simulink model "Control_PID_Senoidal_orientacion"  (R2024b)
settings: Solver=FixedStepAuto  StartTime=0.0  StopTime=30.0  FixedStep=1e-3  RelTol=1e-3
settings Model: Creator=Raul Robles  LastModifiedBy=Raul Robles

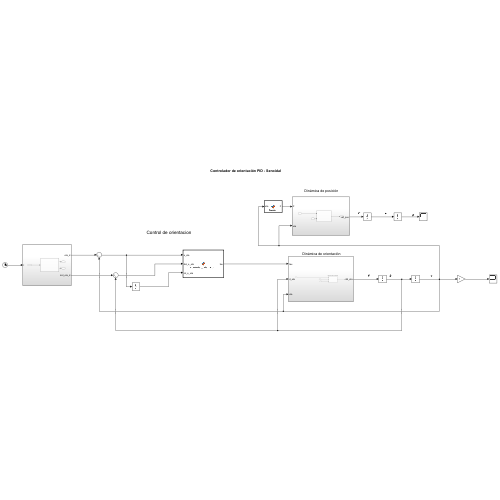
[thumbnail: Simulink's stored preview of the top-level diagram]
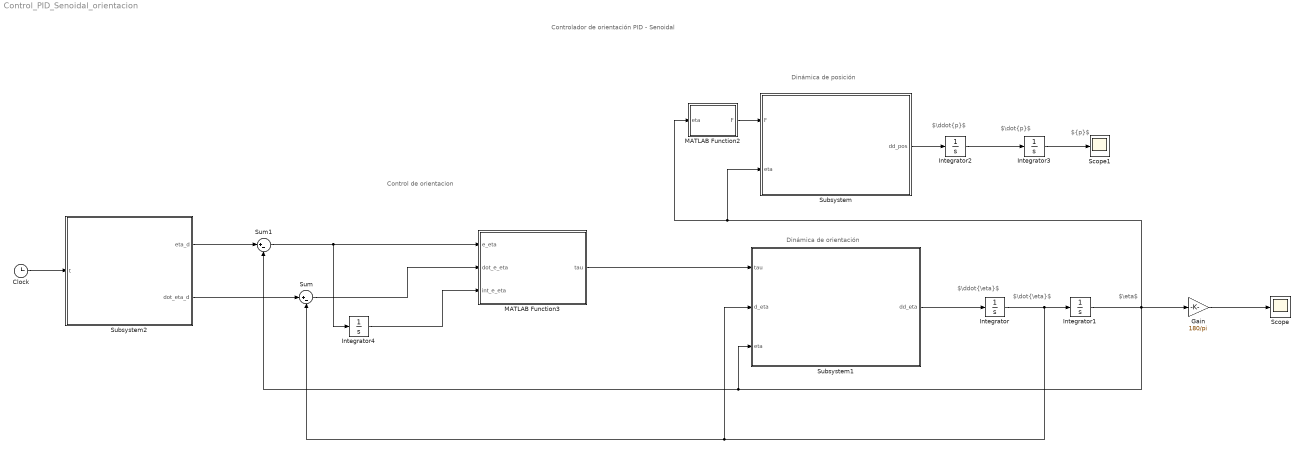
== system Control_PID_Senoidal_orientacion ==
  note: Controlador de orientación PID - Senoidal
  note: $\dot{\eta}$
  note: $\ddot{p}$
  note: $\ddot{\eta}$
  note: Dinámica de posición
  note: ${p}$
  note: $\eta$
  note: Control de orientacion
  note: $\dot{p}$
  note: Dinámica de orientación
  Clock : Clock
      settings: Decimation=30
  Gain : Gain  Gain=180/pi
  Integrator{,1..4} (5 alike) : Integrator  InitialCondition=[0; 0; 0]
  MATLAB Function2 : MATLAB Function  TreatAsAtomicUnit=on
  MATLAB Function3 : MATLAB Function  TreatAsAtomicUnit=on
  Scope : Scope
  Scope1 : Scope
  Subsystem : Subsystem
  Subsystem1 : Subsystem
  Subsystem2 : Subsystem
  Sum : Sum  Inputs=|+-
  Sum1 : Sum  Inputs=|+-
  wires:
  Integrator2/1 -> Integrator3/1
  Integrator3/1 -> Scope1/1
  MATLAB Function2/1(F) -> Subsystem/1(F)
  Subsystem/1(dd_pos) -> Integrator2/1
  Subsystem1/1(dd_eta) -> Integrator/1
  Integrator/1 -> Subsystem1/2(d_eta), Sum/2, Integrator1/1
  Integrator1/1 -> Sum1/2, Subsystem1/3(eta), Gain/1, MATLAB Function2/1(eta), Subsystem/2(eta)
  Gain/1 -> Scope/1
  MATLAB Function3/1(tau) -> Subsystem1/1(tau)
  Clock/1 -> Subsystem2/1(t)
  Subsystem2/1(eta_d) -> Sum1/1
  Subsystem2/2(dot_eta_d) -> Sum/1
  Sum1/1 -> Integrator4/1, MATLAB Function3/1(e_eta)
  Sum/1 -> MATLAB Function3/2(dot_e_eta)
  Integrator4/1 -> MATLAB Function3/3(int_e_eta)

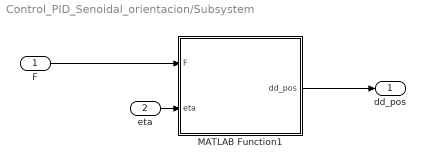
== system Control_PID_Senoidal_orientacion/Subsystem ==
  F : Inport
  eta : Inport  Port=2
  MATLAB Function1 : MATLAB Function  TreatAsAtomicUnit=on
  dd_pos : Outport
  wires:
  MATLAB Function1/1(dd_pos) -> dd_pos/1
  eta/1 -> MATLAB Function1/2(eta)
  F/1 -> MATLAB Function1/1(F)

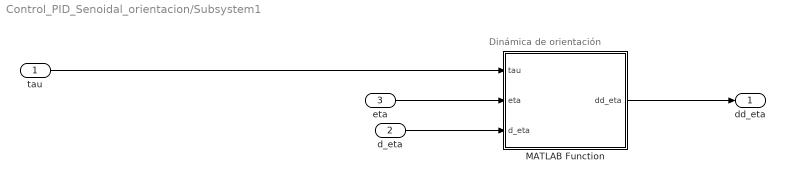
== system Control_PID_Senoidal_orientacion/Subsystem1 ==
  note: Dinámica de orientación
  tau : Inport
  d_eta : Inport  Port=2
  eta : Inport  Port=3
  MATLAB Function : MATLAB Function  TreatAsAtomicUnit=on
  dd_eta : Outport
  wires:
  d_eta/1 -> MATLAB Function/3(d_eta)
  eta/1 -> MATLAB Function/2(eta)
  MATLAB Function/1(dd_eta) -> dd_eta/1
  tau/1 -> MATLAB Function/1(tau)

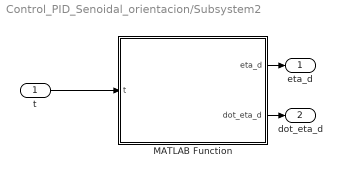
== system Control_PID_Senoidal_orientacion/Subsystem2 ==
  t : Inport
  MATLAB Function : MATLAB Function  TreatAsAtomicUnit=on
  eta_d : Outport
  dot_eta_d : Outport  Port=2
  wires:
  t/1 -> MATLAB Function/1(t)
  MATLAB Function/2(dot_eta_d) -> dot_eta_d/1
  MATLAB Function/1(eta_d) -> eta_d/1

== matlab function Control_PID_Senoidal_orientacion/Subsystem1/MATLAB Function ==
  data: tau input; dd_eta output; eta input; d_eta input
function dd_eta = orientation_dynamics(tau, eta, d_eta)
    
    % Matriz de inercia (momento de inercia)
    Ixx = 0.00273;
    Iyy = 0.00273;
    Izz = 0.00541;
    I = diag([Ixx, Iyy, Izz]);

    % Matriz de transformación PHI
    PHI_11 = 1;
    PHI_12 = sin(eta(1))*tan(eta(2));
    PHI_13 = cos(eta(1))*tan(eta(2));
    PHI_21 = 0;
    PHI_22 = cos(eta(1));
    PHI_23 = -sin(eta(1));
    PHI_31 = 0;
    PHI_32 = sin(eta(1))/cos(eta(2));
    PHI_33 = cos(eta(1))/cos(eta(2));

    PHI = [
        PHI_11, PHI_12, PHI_13;
        PHI_21, PHI_22, PHI_23;
        PHI_31, PHI_32, PHI_33
    ];
    
    % Derivada de la matriz PHI
    PHI_D_11 = 0;
    PHI_D_12 = d_eta(1)*cos(eta(1))*tan(eta(2)) + d_eta(2)*(sin(eta(1))/(cos(eta(2))^2));
    PHI_D_13 = d_eta(2)*(cos(eta(1))/(cos(eta(2))^2)) - d_eta(1)*sin(eta(1))*tan(eta(2));
    PHI_D_21 = 0;
    PHI_D_22 = -d_eta(1)*sin(eta(1));
    PHI_D_23 = -d_eta(1)*cos(eta(1));
    PHI_D_31 = 0;
    PHI_D_32 = (cos(eta(1))*cos(eta(2))*d_eta(1) + sin(eta(1))*sin(eta(2))*d_eta(2))/(cos(eta(2))^2);
    PHI_D_33 = (cos(eta(1))*sin(eta(2))*d_eta(2) - sin(eta(1))*cos(eta(2))*d_eta(1))/(cos(eta(2))^2);
    
    PHI_D = [
        PHI_D_11, PHI_D_12, PHI_D_13;
        PHI_D_21, PHI_D_22, PHI_D_23;
        PHI_D_31, PHI_D_32, PHI_D_33
    ];
    
   
    PHI_inv = inv(PHI); %%Inversa de la matriz PHI
    M = (PHI_inv') * I * PHI_inv; %%% Matriz M
    M_1 = inv(M); %%Inversa de la matriz M
    
    % Matriz S
    S = [0 -1 1; 1 0 -1; -1 1 0];
    
    % Matriz Coriolis
    C = (PHI_inv') * (S * (I * (PHI_inv)) - I * (PHI_inv) * PHI_D) * PHI_inv;
    
    fn = (PHI_inv') * tau; 

    % Cálculo de la aceleración angular
    dd_eta = (M_1) * (-C * d_eta + fn);
end

== matlab function Control_PID_Senoidal_orientacion/MATLAB Function2 ==
  data: eta input; F output
function F = fuerza(eta)

%%% Masa del quad
m = 0.8;
%%% Gravedad
g = 9.81;

F = 1.0002*m*g/(cos(eta(1))*cos(eta(2)));

== matlab function Control_PID_Senoidal_orientacion/MATLAB Function3 ==
  data: e_eta input; tau output; dot_e_eta input; int_e_eta input
function tau = controller_orientation(e_eta,dot_e_eta,int_e_eta)

v1 = [0.9 0.9 0.9];
v2 = [2.2 2.2 2.2];
v3 = [0.15 0.15 0.15];

%%% Ganancias de los controladores

Kp = diag(v1);
Ki = diag(v2);
Kd = diag(v3);


tau = Kp*e_eta + Kd*dot_e_eta + Ki*int_e_eta;

== matlab function Control_PID_Senoidal_orientacion/Subsystem2/MATLAB Function ==
  data: t input; eta_d output; dot_eta_d output
function [eta_d,dot_eta_d] = fcn(t)

%%% Orientaciones deseadas
phi_d = (10*pi/180)*sin((2*pi*t)/30);
theta_d = (10*pi/180)*sin((2*pi*t)/30);
psi_d = (30*pi/180)*sin((2*pi*t)/30);

eta_d = [phi_d; theta_d; psi_d];

%%% Derivada de la orientacion deseada

dot_phi_d = (2*pi/30)*(10*pi/180)*cos((2*pi*t)/30);
dot_theta_d = (2*pi/30)*(10*pi/180)*cos((2*pi*t)/30);
dot_psi_d = (2*pi/30)*(30*pi/180)*cos((2*pi*t)/30);

dot_eta_d = [dot_phi_d; dot_theta_d; dot_psi_d];

== matlab function Control_PID_Senoidal_orientacion/Subsystem/MATLAB Function1 ==
  data: F input; dd_pos output; eta input
function dd_pos = position_dynamics(F, eta)
    
%%% Masa del quad
m = 0.8; %%%[kg]

%%% Vector de gravedad
g = 9.81;
gz = [0; 0; g];

%%% Matriz de rotacion

R_11 = cos(eta(2))*cos(eta(3));
R_12 = sin(eta(1))*sin(eta(2))*cos(eta(3)) - cos(eta(1))*sin(eta(3));
R_13 = cos(eta(1))*sin(eta(2))*cos(eta(3)) + sin(eta(1))*sin(eta(3));
R_21 = cos(eta(2))*sin(eta(3));
R_22 = sin(eta(1))*sin(eta(2))*sin(eta(3)) + cos(eta(1))*cos(eta(3));
R_23 = cos(eta(1))*sin(eta(2))*sin(eta(3)) - sin(eta(1))*cos(eta(3));
R_31 = -sin(eta(2));
R_32 = sin(eta(1))*cos(eta(2));
R_33 = cos(eta(1))*cos(eta(2));

R = [R_11 R_12 R_13; R_21 R_22 R_23; R_31 R_32 R_33];

%%%% Vector r3

r3 = R*[0; 0; 1];

%%% Vector fp (fuerza en el marco de referencia inercial)

fp = r3*F;
% Dinámica de la posición
    dd_pos = (1/m)*fp - gz;
end
